simulink subsystem "input_muxer"  (R2021a)
settings: Solver=VariableStepAuto  StartTime=0.0  StopTime=10.0  RelTol=1e-3
libraries: hdlBasic x13
settings Model: Creator=ckk5  LastModifiedBy=ckk5

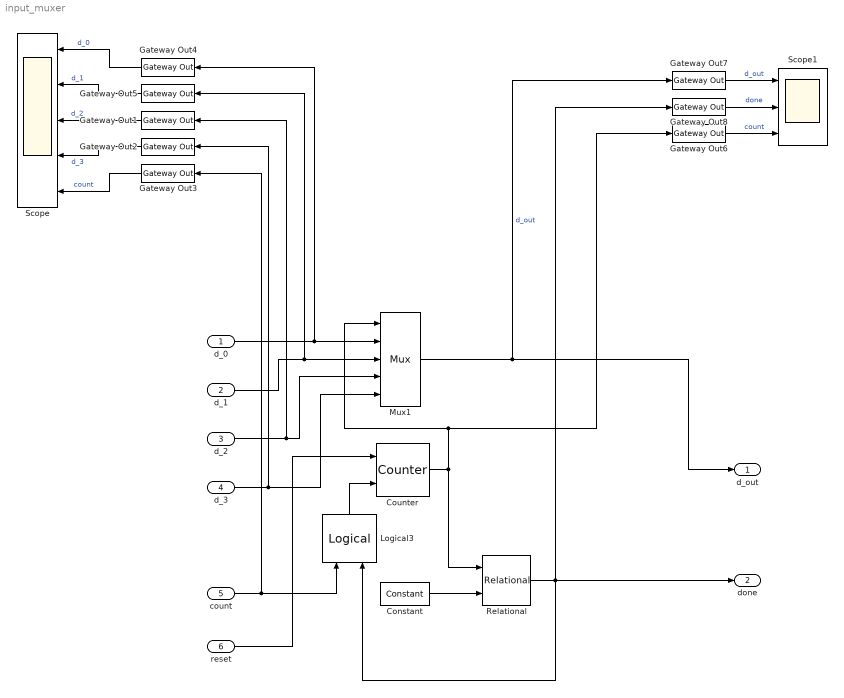
== system input_muxer ==
  d_0 : Inport
  d_1 : Inport  Port=2
  d_2 : Inport  Port=3
  d_3 : Inport  Port=4
  count : Inport  Port=5
  reset : Inport  Port=6
  Constant : hdlBasic/Constant  const=3  gui_display_data_type=Fixed-point  arith_type=Unsigned  n_bits=2  bin_pt=0  preci_type=Single  exp_width=8  frac_width=24  explicit_period=off  period=1  XmcBlockStatus=1  maskContainerNames=tabcontainer1  block_type=constant  block_config=sysgen:Constant_config
  Counter : hdlBasic/Counter  cnt_type=Count limited  cnt_to=3  operation=Up  start_count=0  cnt_by_val=1  arith_type=Unsigned  n_bits=2  bin_pt=0  load_pin=off  rst=on  en=on  explicit_period=Explicit  period=1  use_behavioral_HDL=off  implementation=Fabric  XmcBlockStatus=1  maskContainerNames=group1  block_type=counter  block_config=sysgen:Counter_config
  Gateway Out{1..8} (8 alike) : hdlBasic/Gateway Out  inherit_from_input=off  hdl_port=off  rows=1  columns=1  UseAsDAC=off  DACChannel='1'  interface=None  automatic_assignment=on  address_offset=hex2dec('00')  intf_name=''  intf_description=''  timing_constraint=None  locs_specified=off  LOCs={}  io_standard={}  XmcBlockStatus=1  maskContainerNames=group4  block_type=gatewayout  block_config=sysgen:gateway_out_config  block_width_w=590  block_height_w=620  block_width=620  block_height=750
  Logical3 : hdlBasic/Logical  logical_function=AND  inputs=2  en=off  latency=0  precision=Full  arith_type=Unsigned  n_bits=16  bin_pt=0  align_bp=on  overflow=[]  quantization=[]  XmcBlockStatus=1  maskContainerNames=tabcontainer1  block_type=logical  block_config=sysgen:Logical_config
  Mux1 : hdlBasic/Mux  inputs=4  en=off  latency=0  precision=Full  arith_type=Unsigned  n_bits=16  bin_pt=14  quantization=Truncate  overflow=Wrap  XmcBlockStatus=1  maskContainerNames=tabcontainer1  block_type=mux  block_config=sysgen:Mux_config
  Relational : hdlBasic/Relational  mode=a!=b  op_type=Bool  en=off  latency=0  XmcBlockStatus=1  maskContainerNames=tabcontainer1  block_type=relational  block_config=sysgen:Relational_config
  Scope : Scope  NumInputPorts=5
  Scope1 : Scope  NumInputPorts=3
  d_out : Outport
  done : Outport  Port=2
  wires:
  d_2/1 -> Mux1/4, Gateway Out1/1
  Counter/1 -> Relational/1, Gateway Out6/1, Mux1/1
  d_0/1 -> Mux1/2, Gateway Out4/1
  d_3/1 -> Mux1/5, Gateway Out2/1
  d_1/1 -> Mux1/3, Gateway Out5/1
  Mux1/1 -> d_out/1, Gateway Out7/1  "d_out"
  Logical3/1 -> Counter/2
  Relational/1 -> done/1, Gateway Out8/1, Logical3/2
  Constant/1 -> Relational/2
  count/1 -> Logical3/1, Gateway Out3/1
  Gateway Out4/1 -> Scope/1  "d_0"
  Gateway Out5/1 -> Scope/2  "d_1"
  Gateway Out1/1 -> Scope/3  "d_2"
  Gateway Out2/1 -> Scope/4  "d_3"
  Gateway Out3/1 -> Scope/5  "count"
  Gateway Out7/1 -> Scope1/1  "d_out"
  Gateway Out8/1 -> Scope1/2  "done"
  Gateway Out6/1 -> Scope1/3  "count"
  reset/1 -> Counter/1
